simulink model "Filtro_compensa_CIC"  (R2018a)
settings: Solver=VariableStepAuto  StartTime=0.0  StopTime=2e-3  RelTol=1e-3  EnableMultiTasking=on
values from neighbouring files (symbols this model uses):
  fo = 15000    [Param_compensaCIC.m]
  fs = 50000    [Param_compensaCIC.m]
  Win = 16    [Param_compensaCIC.m]
libraries: dspsrcs4 x3
settings Model: Creator=asperez  LastModifiedBy=damares
settings OptimizationCC: LifeSpan=inf
settings DebuggingCC: LibraryContextMissingDiagnostic=warning  SFUnexpectedBacktrackingDiag=warning  SFNoUnconditionalDefaultTransitionDiag=warning
settings CodeAppCC: StateflowObjectComments=on
settings GRTTargetCC: TargetLangStandard=C89/C90 (ANSI)  GeneratePreprocessorConditionals=Disable all
settings ConfigComp: CovMetricSettings=dw  CovHtmlReporting=on  CovSaveCumulativeToWorkspaceVar=on  CovSaveSingleToWorkspaceVar=on  CovExternalEMLEnable=off

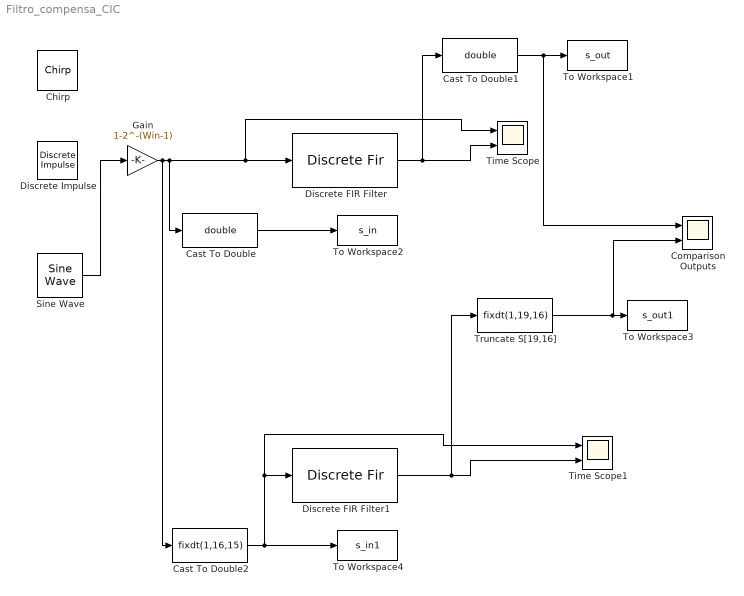
== system Filtro_compensa_CIC ==
  Cast To Double : DataTypeConversion  OutDataTypeStr=double
  Cast To Double1 : DataTypeConversion  OutDataTypeStr=double
  Cast To Double2 : DataTypeConversion  OutDataTypeStr=fixdt(1,16,15)
  Chirp : dspsrcs4/Chirp  sweep=Linear  mode=Unidirectional  f0=1000  f1=4000  t1=1  Tsweep=1  phase=0  Ts=1/8000  spf=1  datatype=Double  OutputFrames=off
      settings: SourceProductName=DSP System Toolbox
  "Comparison Outputs " : Scope  NumInputPorts=2
  Discrete Impulse : dspsrcs4/Discrete  Impulse  Delay=0  SampleTime=1/fs  FrameSample=1  OutputFrames=off  dataType=double  isSigned=on  wordLen=16  udDataType=sfix(16)  fracBitsMode=User-defined  numFracBits=15  OutDataTypeStr=double  LastOutDataTypeStr=double
  Discrete FIR Filter : DiscreteFir  Coefficients=h_q'  OutDataTypeStr=Inherit: Same as input
  Discrete FIR Filter1 : DiscreteFir  Coefficients=h_q'  CoefDataTypeStr=fixdt(1,18,16)  ProductDataTypeStr=fixdt(1,34,32)  AccumDataTypeStr=fixdt(1,38,32)  OutDataTypeStr=fixdt(1,38,32)
  Gain : Gain  Gain=1-2^-(Win-1)  OutDataTypeStr=double
  Sine Wave : dspsrcs4/Sine Wave  Amplitude=1  Frequency=fo  Phase=0  SampleMode=Discrete  OutComplex=Real  CompMethod=Trigonometric fcn  TableSize=Speed  SampleTime=1/fs  SamplesPerFrame=1  ResetState=Restart at time zero  OutputFrames=off  dataType=double  wordLen=16  udDataType=sfix(16)  fracBitsMode=User-defined  numFracBits=14  OutDataTypeStr=double  LastOutDataTypeStr=double
  Time Scope : Scope  NumInputPorts=2
  Time Scope1 : Scope  NumInputPorts=2
  To Workspace1 : ToWorkspace  VariableName=s_out  SampleTime=-1
  To Workspace2 : ToWorkspace  VariableName=s_in  SampleTime=-1
      settings: Save2DSignal=2-D array (concatenate along first dimension)
  To Workspace3 : ToWorkspace  VariableName=s_out1  SampleTime=-1
  To Workspace4 : ToWorkspace  VariableName=s_in1  SampleTime=-1
      settings: Save2DSignal=2-D array (concatenate along first dimension)
  Truncate S[19,16] : DataTypeConversion  OutDataTypeStr=fixdt(1,19,16)
  wires:
  Discrete FIR Filter/1 -> Cast To Double1/1, Time Scope/2
  Sine Wave/1 -> Gain/1
  Cast To Double/1 -> To Workspace2/1
  Cast To Double1/1 -> "Comparison Outputs "/1, To Workspace1/1
  Cast To Double2/1 -> Discrete FIR Filter1/1, Time Scope1/1, To Workspace4/1
  Discrete FIR Filter1/1 -> Time Scope1/2, Truncate S[19,16]/1
  Gain/1 -> Cast To Double2/1, Cast To Double/1, Time Scope/1, Discrete FIR Filter/1
  Truncate S[19,16]/1 -> "Comparison Outputs "/2, To Workspace3/1
